simulink model "Hopper_lqr"  (R2024b)
settings: Solver=VariableStepAuto  StartTime=0.0  StopTime=60.0  RelTol=1e-3
values from neighbouring files (symbols this model uses):
  eta = [0.6, 0.6, 10]    [LinearStateSpace.m]
  K = Kd(:,1:10)    [LinearStateSpace.m]
  Kf = -(Cred*((Ared-Bred*K)\Bred))\eye(3)    [LinearStateSpace.m]
  Ki = Kd(:,11:13)    [LinearStateSpace.m]
  params = [mval; mdotval; Iaval; Iadotval; Izzval; Izzdotval; lzval]    [LinearStateSpace.m]
  Teq = double(subs(ueq(1), [m; g], [mval; gval]))    [LinearStateSpace.m]
  Ts = 0.005    [LinearStateSpace.m]
undefined symbols (not defined in the file or in its folder): DiscIntNeverNeededParam
libraries: simulink x2
settings Model: Creator=Yusuf  LastModifiedBy=Yusuf

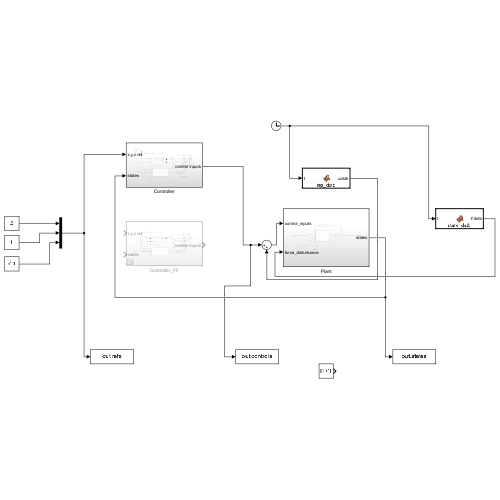
[thumbnail: Simulink's stored preview of the top-level diagram]
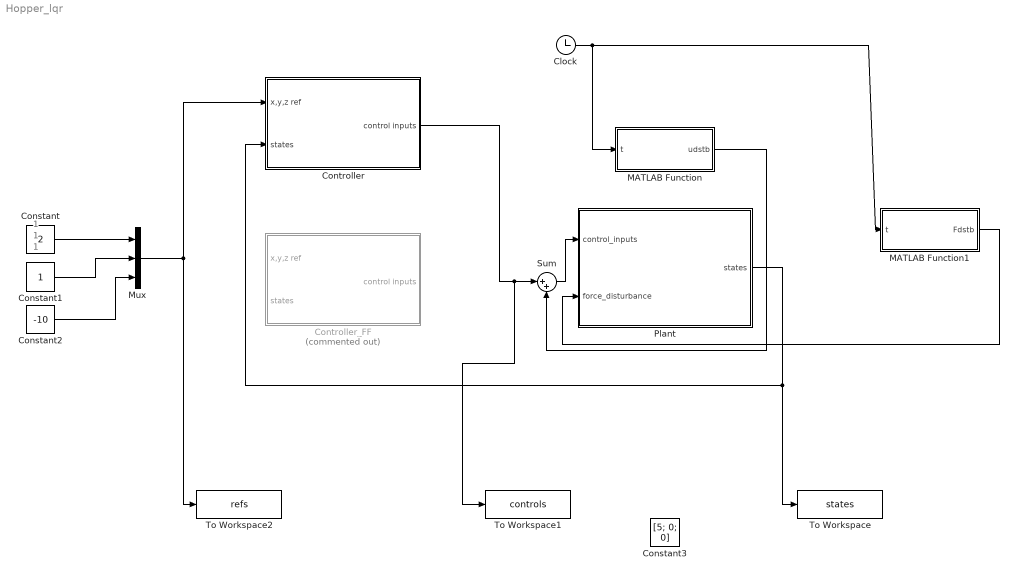
== system Hopper_lqr ==
  note: 1
  note: 1
  note: 1
  Clock : Clock
  Constant : Constant  Value=2  SampleTime=Ts
  Constant1 : Constant  SampleTime=Ts
  Constant2 : Constant  Value=-10  SampleTime=Ts
  Constant3 : Constant  Value=[5; 0; 0]
  Controller : Subsystem
  Controller_FF : Subsystem  Commented=on
  MATLAB Function : MATLAB Function  TreatAsAtomicUnit=on
  MATLAB Function1 : MATLAB Function  TreatAsAtomicUnit=on
  Mux : Mux  Inputs=3
  Plant : Subsystem
  Sum : Sum  Inputs=|++
  To Workspace : ToWorkspace  VariableName=states  SaveFormat=Structure With Time  SampleTime=-1
  To Workspace1 : ToWorkspace  VariableName=controls  SaveFormat=Structure With Time  SampleTime=-1
  To Workspace2 : ToWorkspace  VariableName=refs  SaveFormat=Structure With Time  SampleTime=-1
  wires:
  Mux/1 -> Controller/1(x,y,z ref), To Workspace2/1
  Constant/1 -> Mux/1
  Constant1/1 -> Mux/2
  Constant2/1 -> Mux/3
  Plant/1(states) -> Controller/2(states), To Workspace/1
  Controller/1(control inputs) -> To Workspace1/1, Sum/1
  Sum/1 -> Plant/1(control_inputs)
  Clock/1 -> MATLAB Function/1(t), MATLAB Function1/1(t)
  MATLAB Function/1(udstb) -> Sum/2
  MATLAB Function1/1(Fdstb) -> Plant/2(force_disturbance)

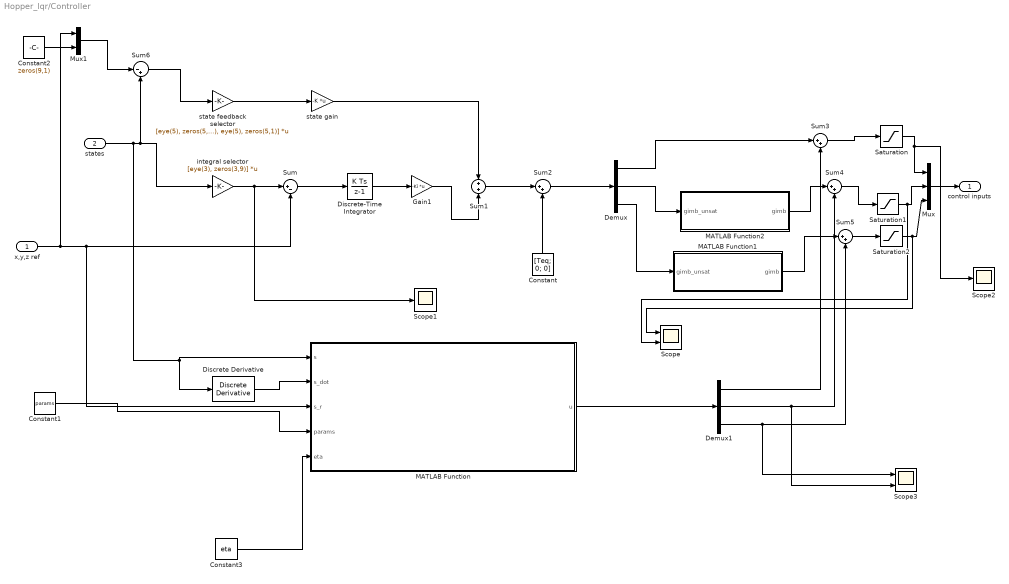
== system Hopper_lqr/Controller ==
  x,y,z ref : Inport
  states : Inport  Port=2
  Constant : Constant  Value=[Teq; 0; 0]  SampleTime=Ts
  Constant1 : Constant  Value=params
  Constant2 : Constant  Value=zeros(9,1)
  Constant3 : Constant  Value=eta
  Demux : Demux  Outputs=3
  Demux1 : Demux  Outputs=3
  Discrete Derivative : simulink/Discrete/Discrete Derivative  gainval=1.0  ICPrevScaledInput=0.0  OutMin=[]  OutMax=[]  OutDataType=fixdt(1, 16)  OutScaling=2^-10  DoSatur=off
  Discrete-Time Integrator : DiscreteIntegrator  SampleTime=Ts  ICPrevOutput=DiscIntNeverNeededParam  ICPrevScaledInput=DiscIntNeverNeededParam
  Gain1 : Gain  Gain=-Ki  Multiplication=Matrix(K*u)
  MATLAB Function : MATLAB Function  TreatAsAtomicUnit=on
  MATLAB Function1 : MATLAB Function  TreatAsAtomicUnit=on
  MATLAB Function2 : MATLAB Function  TreatAsAtomicUnit=on
  Mux : Mux  Inputs=3
  Mux1 : Mux  Inputs=2
  Saturation : Saturate  UpperLimit=500  LowerLimit=0
  Saturation1 : Saturate  UpperLimit=pi/6  LowerLimit=-pi/6
  Saturation2 : Saturate  UpperLimit=pi/6  LowerLimit=-pi/6
  Scope : Scope  NumInputPorts=2
  Scope1 : Scope
  Scope2 : Scope
  Scope3 : Scope  NumInputPorts=2
  Sum : Sum  Inputs=|+-
  Sum1 : Sum
  Sum{2..5} (4 alike) : Sum  Inputs=|++
  Sum6 : Sum  Inputs=|-+
  integral selector : Gain  Gain=[eye(3), zeros(3,9)]  Multiplication=Matrix(K*u)
  state feedback selector : Gain  Gain=[eye(5), zeros(5,7); zeros(5,6), eye(5), zeros(5,1)]  Multiplication=Matrix(K*u)
  state gain : Gain  Gain=-K  Multiplication=Matrix(K*u)
  control inputs : Outport
  wires:
  integral selector/1 -> Scope1/1, Sum/1
  Constant/1 -> Sum2/2
  Discrete-Time Integrator/1 -> Gain1/1
  state gain/1 -> Sum1/1
  Sum1/1 -> Sum2/1
  state feedback selector/1 -> state gain/1
  Sum/1 -> Discrete-Time Integrator/1
  states/1 -> Sum6/2, integral selector/1, Discrete Derivative/1, MATLAB Function/1(s)
  x,y,z ref/1 -> MATLAB Function/3(s_r), Sum/2, Mux1/1
  Gain1/1 -> Sum1/2
  Constant1/1 -> MATLAB Function/4(params)
  Discrete Derivative/1 -> MATLAB Function/2(s_dot)
  MATLAB Function/1(u) -> Demux1/1
  Sum2/1 -> Demux/1
  Mux/1 -> control inputs/1
  Demux1/1 -> Sum3/2
  Demux1/2 -> Scope3/2, Sum4/2
  Demux1/3 -> Scope3/1, Sum5/2
  Demux/2 -> MATLAB Function2/1(gimb_unsat)
  Demux/3 -> MATLAB Function1/1(gimb_unsat)
  Sum4/1 -> Saturation1/1
  Sum5/1 -> Saturation2/1
  Demux/1 -> Sum3/1
  Sum3/1 -> Saturation/1
  Saturation/1 -> Scope2/1, Mux/1
  MATLAB Function2/1(gimb) -> Sum4/1
  MATLAB Function1/1(gimb) -> Sum5/1
  Saturation2/1 -> Scope/1, Mux/3
  Saturation1/1 -> Scope/2, Mux/2
  Constant2/1 -> Mux1/2
  Mux1/1 -> Sum6/1
  Sum6/1 -> state feedback selector/1
  Constant3/1 -> MATLAB Function/5(eta)

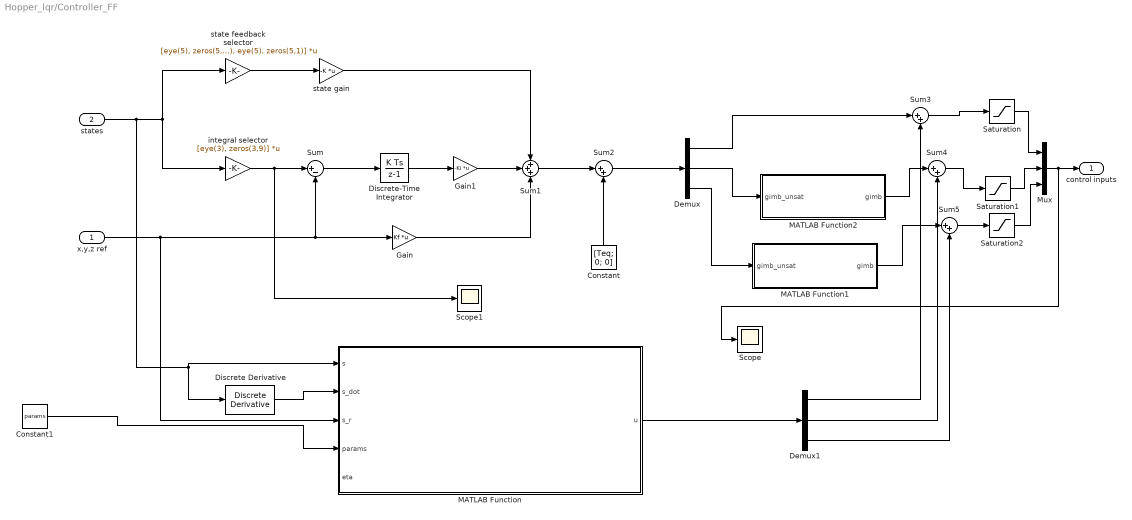
== system Hopper_lqr/Controller_FF ==
  x,y,z ref : Inport
  states : Inport  Port=2
  Constant : Constant  Value=[Teq; 0; 0]  SampleTime=Ts
  Constant1 : Constant  Value=params
  Demux : Demux  Outputs=3
  Demux1 : Demux  Outputs=3
  Discrete Derivative : simulink/Discrete/Discrete Derivative  gainval=1.0  ICPrevScaledInput=0.0  OutMin=[]  OutMax=[]  OutDataType=fixdt(1, 16)  OutScaling=2^-10  DoSatur=off
  Discrete-Time Integrator : DiscreteIntegrator  SampleTime=Ts  ICPrevOutput=DiscIntNeverNeededParam  ICPrevScaledInput=DiscIntNeverNeededParam
  Gain : Gain  Gain=Kf  Multiplication=Matrix(K*u)
  Gain1 : Gain  Gain=-Ki  Multiplication=Matrix(K*u)
  MATLAB Function : MATLAB Function  TreatAsAtomicUnit=on
  MATLAB Function1 : MATLAB Function  TreatAsAtomicUnit=on
  MATLAB Function2 : MATLAB Function  TreatAsAtomicUnit=on
  Mux : Mux  Inputs=3
  Saturation : Saturate  UpperLimit=50  LowerLimit=0
  Saturation1 : Saturate  UpperLimit=pi/6  LowerLimit=-pi/6
  Saturation2 : Saturate  UpperLimit=pi/6  LowerLimit=-pi/6
  Scope : Scope
  Scope1 : Scope
  Sum : Sum  Inputs=|+-
  Sum1 : Sum  Inputs=+++
  Sum{2..5} (4 alike) : Sum  Inputs=|++
  integral selector : Gain  Gain=[eye(3), zeros(3,9)]  Multiplication=Matrix(K*u)
  state feedback selector : Gain  Gain=[eye(5), zeros(5,7); zeros(5,6), eye(5), zeros(5,1)]  Multiplication=Matrix(K*u)
  state gain : Gain  Gain=-K  Multiplication=Matrix(K*u)
  control inputs : Outport
  wires:
  integral selector/1 -> Scope1/1, Sum/1
  Constant/1 -> Sum2/2
  Discrete-Time Integrator/1 -> Gain1/1
  state gain/1 -> Sum1/1
  Sum1/1 -> Sum2/1
  state feedback selector/1 -> state gain/1
  Sum/1 -> Discrete-Time Integrator/1
  states/1 -> Discrete Derivative/1, MATLAB Function/1(s), integral selector/1, state feedback selector/1
  Gain/1 -> Sum1/3
  x,y,z ref/1 -> MATLAB Function/3(s_r), Sum/2, Gain/1
  Gain1/1 -> Sum1/2
  Constant1/1 -> MATLAB Function/4(params)
  Discrete Derivative/1 -> MATLAB Function/2(s_dot)
  MATLAB Function/1(u) -> Demux1/1
  Sum2/1 -> Demux/1
  Mux/1 -> Scope/1, control inputs/1
  Demux1/1 -> Sum3/2
  Demux1/2 -> Sum4/2
  Demux1/3 -> Sum5/2
  Demux/2 -> MATLAB Function2/1(gimb_unsat)
  Demux/3 -> MATLAB Function1/1(gimb_unsat)
  Sum4/1 -> Saturation1/1
  Sum5/1 -> Saturation2/1
  Demux/1 -> Sum3/1
  Sum3/1 -> Saturation/1
  Saturation/1 -> Mux/1
  MATLAB Function2/1(gimb) -> Sum4/1
  MATLAB Function1/1(gimb) -> Sum5/1
  Saturation2/1 -> Mux/3
  Saturation1/1 -> Mux/2

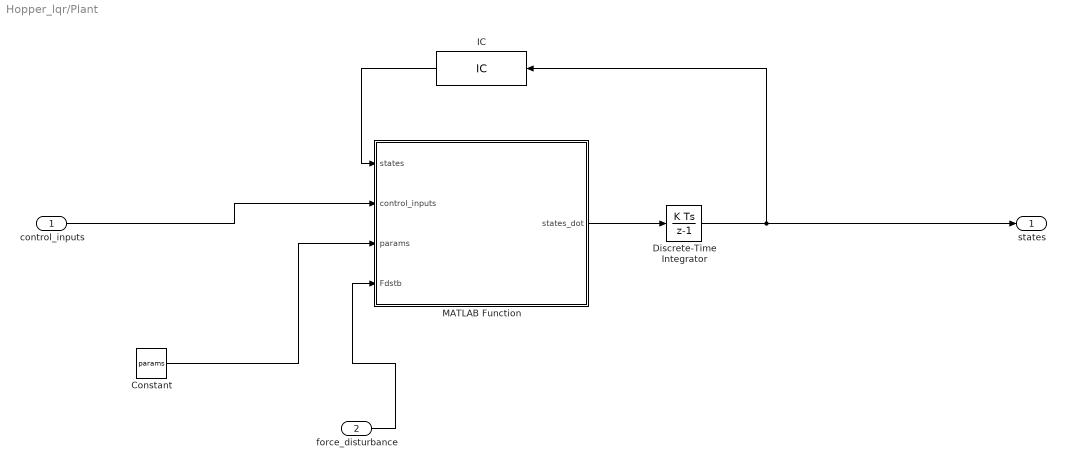
== system Hopper_lqr/Plant ==
  control_inputs : Inport
  force_disturbance : Inport  Port=2
  Constant : Constant  Value=params
  Discrete-Time Integrator : DiscreteIntegrator  SampleTime=-1  ICPrevOutput=DiscIntNeverNeededParam  ICPrevScaledInput=DiscIntNeverNeededParam
  IC : InitialCondition  Value=zeros(12,1)
  MATLAB Function : MATLAB Function  TreatAsAtomicUnit=on
  states : Outport
  wires:
  Constant/1 -> MATLAB Function/3(params)
  control_inputs/1 -> MATLAB Function/2(control_inputs)
  Discrete-Time Integrator/1 -> states/1, IC/1
  MATLAB Function/1(states_dot) -> Discrete-Time Integrator/1
  IC/1 -> MATLAB Function/1(states)
  force_disturbance/1 -> MATLAB Function/4(Fdstb)

== matlab function Hopper_lqr/Controller_FF/MATLAB Function ==
  data: s input; s_dot input; s_r input; params input; u output; eta input
function u = SMC(s, s_dot, s_r, params, eta)
% rocketController - Backstepping-based + Sliding Mode Control for rocket dynamics

m = params(1);

% Constants
g = 9.81; % Gravity

% Extract current statestates
x = s(1);
y = s(2);
z = s(3);
x_dot = s_dot(1);
y_dot = s_dot(2);
z_dot = s_dot(3);

% Extract reference states
x_ref = s_r(1);
y_ref = s_r(2);
z_ref = s_r(3);
x_dot_ref = 0;
y_dot_ref = 0;
z_dot_ref = 0;

% Sliding Mode Gains
lambda_x = 0.1;  % Tuning parameter for x sliding surface
lambda_z = 0.1;  % Tuning parameter for z sliding surface
lambda_y = 0.1;  % Tuning parameter for theta sliding surface

eta_x = eta(1); eta_y = eta(2); eta_z = eta(3);

psi_x = 1;
psi_z = 1;
psi_y = 1;

% Define Sliding Surfaces
ex = x - x_ref;
ez = z - z_ref;
ey = y - y_ref;
edotx = x_dot - x_dot_ref;
edotz = z_dot - z_dot_ref;
edoty = y_dot - y_dot_ref;

sx = edotx + lambda_x * ex;  % Sliding surface for x
sy = edoty + lambda_y * ey;  % Sliding surface for x
sz = edotz + lambda_z * ez;  % Sliding surface for z

% Smooth Sliding Mode Control (Using Tanh Function)
SMC_x = -eta_x * tanh(sx / psi_x);
SMC_y = -eta_y * tanh(sy / psi_y);
SMC_z = -eta_z * tanh(sz / psi_z);

% Desired acceleration (Modified with SMC)
ax = SMC_x;
ay = SMC_y;
az = SMC_z;

% Compute control inputs
%T = m * sqrt(ax^2 + ay^2 + (az + g)^2); 
Tx = m*ax;
Ty = m*ay;
Tz = m*(az+g);

% Tz = -T*cos(alpha)*cos(beta)
% Ty = T*cos(alpha)*sin(beta)
% Tx = T*sin(alpha)

phi = s(4); theta = s(5); psi = s(6);

T_etob=[cos(theta)*cos(psi), sin(theta)*sin(phi)*cos(psi)-cos(phi)*sin(psi), cos(phi)*sin(theta)*cos(psi)+sin(phi)*sin(psi);
    cos(theta)*sin(psi), sin(phi)*sin(theta)*sin(psi)+cos(phi)*cos(psi), cos(phi)*sin(theta)*sin(psi)-sin(phi)*cos(psi);
    -sin(theta),sin(phi)*cos(theta), cos(phi)*cos(theta)]';

% Compute velocity in inertial frame
Tb=T_etob*[Tx;Ty;Tz];

beta = atan(-Tb(2)/Tb(3));
alpha = atan(Tb(1)/Tb(2)*sin(beta));
T = Tb(1)/sin(alpha);

% Output control vector
u = [T; alpha; beta];

end

== matlab function Hopper_lqr/Plant/MATLAB Function ==
  data: states input; control_inputs input; states_dot output; params input; Fdstb input
function states_dot = state_func(states, control_inputs, params, Fdstb)

g = 9.81;

Fx_d = Fdstb(1);
Fy_d = Fdstb(2);
Fz_d = Fdstb(3);

m = params(1);
mdot = params(2);
Ia = params(3);
Iadot = params(4);
Izz = params(5);
Izzdot = params(6);
lz = params(7);

%%% MASS UNC ----

m = m*1.2;

%%% ------------

x = states(1);
y = states(2);
z = states(3);
phi = states(4);
theta = states(5);
psi = states(6);
U = states(7);
V = states(8);
W = states(9);
p = states(10);
q = states(11);
r = states(12);

T = control_inputs(1);
alpha = control_inputs(2);
beta = control_inputs(3);

Udot = 1/m*(m*(V*r-W*q)-mdot*U-m*g*sin(theta)-T*sin(alpha)+Fx_d);
Vdot = 1/m*(m*(W*p-U*r)-mdot*V+m*g*cos(theta)*sin(phi)+T*cos(alpha)*sin(beta)+Fy_d);
Wdot = 1/m*(m*(U*q-V*p)-mdot*W+m*g*cos(theta)*cos(phi)-T*cos(alpha)*cos(beta)+Fz_d);
pdot = 1/Ia*(-lz*T*cos(alpha)*sin(beta)-q*r*(Izz-Ia)-Iadot*p);
qdot = 1/Ia*(-lz*T*sin(alpha)-r*p*(Ia-Izz)-Iadot*q);
rdot = -Izzdot*r/Izz;

T1 = [1, sin(phi)*tan(theta), cos(phi)*tan(theta);
      0, cos(phi)           , -sin(phi)          ;
      0, sin(phi)*sec(theta), cos(phi)*sec(theta)];

eulerdot = T1*[p;q;r];

T2 = [cos(theta)*cos(psi), -cos(phi)*sin(psi)+sin(phi)*sin(theta)*cos(psi), sin(phi)*sin(psi)+cos(phi)*sin(theta)*cos(psi);
      cos(theta)*sin(psi), cos(phi)*cos(psi)+sin(phi)*sin(theta)*sin(psi) , -sin(phi)*cos(psi)+cos(phi)*sin(theta)*sin(psi);
      -sin(theta)        , sin(phi)*cos(theta)                            , cos(phi)*cos(theta)];

positiondot = T2*[U;V;W];

states_dot = [positiondot; eulerdot; Udot; Vdot; Wdot; pdot; qdot; rdot];

end

== matlab function Hopper_lqr/Controller_FF/MATLAB Function1 ==
  data: gimb_unsat input; gimb output
function gimb = wrap_gimble(gimb_unsat)

% if gimb_unsat < 2*pi+pi/6 && gimb_unsat > 2*pi-pi/6
%     gimb = gimb_unsat-2*pi;
% elseif gimb_unsat > -2*pi-pi/6 && gimb_unsat < -2*pi+pi/6
%     gimb = gimb_unsat+2*pi;
% elseif gimb_unsat > -2*pi+pi/6 && gimb_unsat < -pi
%     gimb = pi/6;
% elseif gimb_unsat < -2*pi-pi/6
%     gimb =-pi/6;
% elseif gimb_unsat < 2*pi-pi/6 && gimb_unsat > pi
%     gimb = -pi/6;
% elseif gimb_unsat > 2*pi+pi/6
%     gimb = pi/6;
% else
%     gimb = gimb_unsat;
% end

gimb = mod(gimb_unsat+pi, 2*pi) - pi;

end

== matlab function Hopper_lqr/Controller_FF/MATLAB Function2 ==
  data: gimb_unsat input; gimb output
function gimb = wrap_gimble(gimb_unsat)

% if gimb_unsat < 2*pi+pi/6 && gimb_unsat > 2*pi-pi/6
%     gimb = gimb_unsat-2*pi;
% elseif gimb_unsat > -2*pi-pi/6 && gimb_unsat < -2*pi+pi/6
%     gimb = gimb_unsat+2*pi;
% elseif gimb_unsat > -2*pi+pi/6 && gimb_unsat < -pi
%     gimb = pi/6;
% elseif gimb_unsat < -2*pi-pi/6
%     gimb =-pi/6;
% elseif gimb_unsat < 2*pi-pi/6 && gimb_unsat > pi
%     gimb = -pi/6;
% elseif gimb_unsat > 2*pi+pi/6
%     gimb = pi/6;
% else
%     gimb = gimb_unsat;
% end

gimb = mod(gimb_unsat+pi, 2*pi) - pi;

end

== matlab function Hopper_lqr/Controller/MATLAB Function ==
  data: s input; s_dot input; s_r input; params input; u output; eta input
function u = SMC(s, s_dot, s_r, params, eta)
% rocketController - Backstepping-based + Sliding Mode Control for rocket dynamics

m = params(1);

% Constants
g = 9.81; % Gravity

% Extract current statestates
x = s(1);
y = s(2);
z = s(3);
x_dot = s_dot(1);
y_dot = s_dot(2);
z_dot = s_dot(3);

% Extract reference states
x_ref = s_r(1);
y_ref = s_r(2);
z_ref = s_r(3);
x_dot_ref = 0;
y_dot_ref = 0;
z_dot_ref = 0;

% Sliding Mode Gains
lambda_x = 0.1;  % Tuning parameter for x sliding surface
lambda_z = 0.1;  % Tuning parameter for z sliding surface
lambda_y = 0.1;  % Tuning parameter for theta sliding surface

eta_x = eta(1); eta_y = eta(2); eta_z = eta(3);

psi_x = 1;
psi_z = 1;
psi_y = 1;

% Define Sliding Surfaces
ex = x - x_ref;
ez = z - z_ref;
ey = y - y_ref;
edotx = x_dot - x_dot_ref;
edotz = z_dot - z_dot_ref;
edoty = y_dot - y_dot_ref;

sx = edotx + lambda_x * ex;  % Sliding surface for x
sy = edoty + lambda_y * ey;  % Sliding surface for x
sz = edotz + lambda_z * ez;  % Sliding surface for z

% Smooth Sliding Mode Control (Using Tanh Function)
SMC_x = -eta_x * tanh(sx / psi_x);
SMC_y = -eta_y * tanh(sy / psi_y);
SMC_z = -eta_z * tanh(sz / psi_z);

% Desired acceleration (Modified with SMC)
ax = SMC_x;
ay = SMC_y;
az = SMC_z;

% Compute control inputs
%T = m * sqrt(ax^2 + ay^2 + (az + g)^2); 
Tx = m*ax;
Ty = m*ay;
Tz = m*(az+g);

% Tz = -T*cos(alpha)*cos(beta)
% Ty = T*cos(alpha)*sin(beta)
% Tx = T*sin(alpha)

phi = s(4); theta = s(5); psi = s(6);

T_etob=[cos(theta)*cos(psi), sin(theta)*sin(phi)*cos(psi)-cos(phi)*sin(psi), cos(phi)*sin(theta)*cos(psi)+sin(phi)*sin(psi);
    cos(theta)*sin(psi), sin(phi)*sin(theta)*sin(psi)+cos(phi)*cos(psi), cos(phi)*sin(theta)*sin(psi)-sin(phi)*cos(psi);
    -sin(theta),sin(phi)*cos(theta), cos(phi)*cos(theta)]';

% Compute velocity in inertial frame
Tb=T_etob*[Tx;Ty;Tz];

beta = atan(-Tb(2)/Tb(3));
alpha = atan(Tb(1)/Tb(2)*sin(beta));
T = Tb(1)/sin(alpha);

% Output control vector
u = [T; alpha; beta];

end

== matlab function Hopper_lqr/Controller/MATLAB Function1 ==
  data: gimb_unsat input; gimb output
function gimb = wrap_gimble(gimb_unsat)

% if gimb_unsat < 2*pi+pi/6 && gimb_unsat > 2*pi-pi/6
%     gimb = gimb_unsat-2*pi;
% elseif gimb_unsat > -2*pi-pi/6 && gimb_unsat < -2*pi+pi/6
%     gimb = gimb_unsat+2*pi;
% elseif gimb_unsat > -2*pi+pi/6 && gimb_unsat < -pi
%     gimb = pi/6;
% elseif gimb_unsat < -2*pi-pi/6
%     gimb =-pi/6;
% elseif gimb_unsat < 2*pi-pi/6 && gimb_unsat > pi
%     gimb = -pi/6;
% elseif gimb_unsat > 2*pi+pi/6
%     gimb = pi/6;
% else
%     gimb = gimb_unsat;
% end

gimb = mod(gimb_unsat+pi, 2*pi) - pi;

end

== matlab function Hopper_lqr/Controller/MATLAB Function2 ==
  data: gimb_unsat input; gimb output
function gimb = wrap_gimble(gimb_unsat)

% if gimb_unsat < 2*pi+pi/6 && gimb_unsat > 2*pi-pi/6
%     gimb = gimb_unsat-2*pi;
% elseif gimb_unsat > -2*pi-pi/6 && gimb_unsat < -2*pi+pi/6
%     gimb = gimb_unsat+2*pi;
% elseif gimb_unsat > -2*pi+pi/6 && gimb_unsat < -pi
%     gimb = pi/6;
% elseif gimb_unsat < -2*pi-pi/6
%     gimb =-pi/6;
% elseif gimb_unsat < 2*pi-pi/6 && gimb_unsat > pi
%     gimb = -pi/6;
% elseif gimb_unsat > 2*pi+pi/6
%     gimb = pi/6;
% else
%     gimb = gimb_unsat;
% end

gimb = mod(gimb_unsat+pi, 2*pi) - pi;

end

== matlab function Hopper_lqr/MATLAB Function ==
  data: t input; udstb output
function udstb = inp_dstb(t)

T = 5*sin(10*t);
alpha = deg2rad(1)*sin(t);
beta = deg2rad(1)*sin(t);

udstb = [T; alpha; beta];

== matlab function Hopper_lqr/MATLAB Function1 ==
  data: t input; Fdstb output
function Fdstb = state_dstb(t)

if t < 30
    Fx = 0;
else
    Fx = 2;
end

Fy = 0;
Fz = 0;

Fdstb = [Fx; Fy; Fz];
